simulink model "QZSFuzzy"  (R2017a)
settings: Solver=ode23tb  StartTime=0.0  StopTime=.04  MaxStep=5e-6  RelTol=1e-3  EnableMultiTasking=on
libraries: powerlib x34, simulink x6, fuzblock x1
settings Model: Creator=acer  LastModifiedBy=acer
settings DataIOCC: LimitDataPoints=on  SaveFormat=Array
settings OptimizationCC: LifeSpan=inf
settings DebuggingCC: SFUnexpectedBacktrackingDiag=warning  SFNoUnconditionalDefaultTransitionDiag=warning  SFExecutionAtInitializationDiag=none
settings HardwareCC: ProdBitPerPointer=32  ProdBitPerSizeT=32  ProdBitPerPtrDiffT=32  ProdLargestAtomicFloat=None  ProdIntDivRoundTo=Undefined  ProdEndianess=Unspecified  ProdWordSize=32  ProdHWDeviceType=32-bit Generic
settings ModelReferenceCC: PropagateSignalLabelsOutOfModel=off
settings GRTTargetCC: TargetLangStandard=C89/C90 (ANSI)  GeneratePreprocessorConditionals=Disable all
settings ConfigComp: CovMetricSettings=dw  CovHtmlReporting=on  CovSaveCumulativeToWorkspaceVar=on  CovSaveSingleToWorkspaceVar=on  CovExternalEMLEnable=off

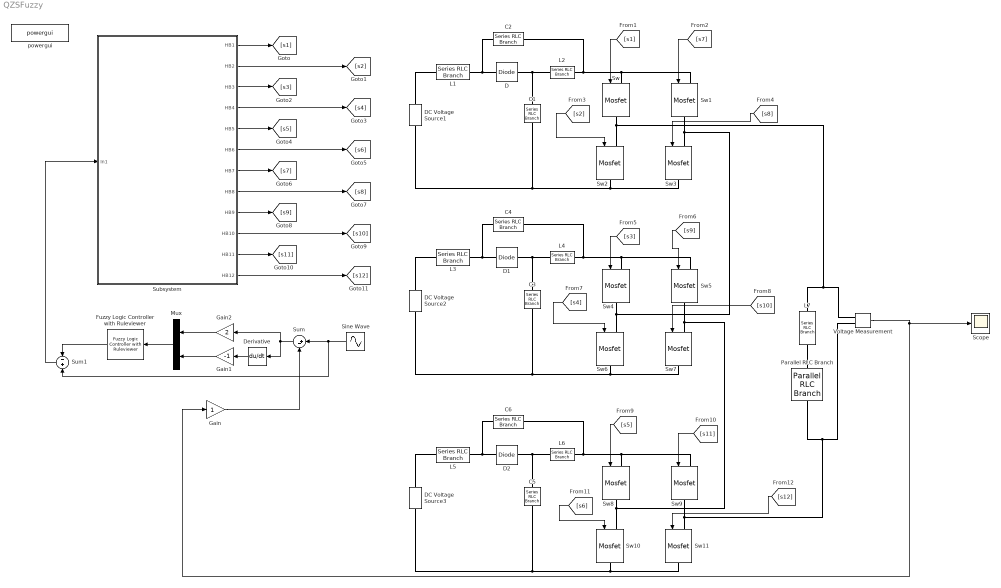
== system QZSFuzzy ==
  C1 : powerlib/Elements/Series RLC Branch  LConnTagsString=__new0  RConnTagsString=__new0  BranchType=C  Resistance=100  Inductance=1e-3  SetiL0=off  InitialCurrent=0  Capacitance=1000e-6  Setx0=off  InitialVoltage=0  Measurements=None
  C2 : powerlib/Elements/Series RLC Branch  LConnTagsString=__new0  RConnTagsString=__new0  BranchType=C  Resistance=1  Inductance=1e-3  SetiL0=off  InitialCurrent=0  Capacitance=1000e-6  Setx0=off  InitialVoltage=0  Measurements=None
  C3 : powerlib/Elements/Series RLC Branch  LConnTagsString=__new0  RConnTagsString=__new0  BranchType=C  Resistance=100  Inductance=1e-3  SetiL0=off  InitialCurrent=0  Capacitance=1000e-6  Setx0=off  InitialVoltage=0  Measurements=None
  C4 : powerlib/Elements/Series RLC Branch  LConnTagsString=__new0  RConnTagsString=__new0  BranchType=C  Resistance=1  Inductance=1e-3  SetiL0=off  InitialCurrent=0  Capacitance=1000e-6  Setx0=off  InitialVoltage=0  Measurements=None
  C5 : powerlib/Elements/Series RLC Branch  LConnTagsString=__new0  RConnTagsString=__new0  BranchType=C  Resistance=100  Inductance=1e-3  SetiL0=off  InitialCurrent=0  Capacitance=1000e-6  Setx0=off  InitialVoltage=0  Measurements=None
  C6 : powerlib/Elements/Series RLC Branch  LConnTagsString=__new0  RConnTagsString=__new0  BranchType=C  Resistance=1  Inductance=1e-3  SetiL0=off  InitialCurrent=0  Capacitance=1000e-6  Setx0=off  InitialVoltage=0  Measurements=None
  D : powerlib/Power Electronics/Diode  Ron=0.001  Lon=0  Vf=.05  IC=0  UseSnubber=off  Rs=500  Cs=250e-9  Measurements=off
  D1 : powerlib/Power Electronics/Diode  Ron=0.001  Lon=0  Vf=.05  IC=0  UseSnubber=off  Rs=500  Cs=250e-9  Measurements=off
  D2 : powerlib/Power Electronics/Diode  Ron=0.001  Lon=0  Vf=.05  IC=0  UseSnubber=off  Rs=500  Cs=250e-9  Measurements=off
  DC Voltage Source1 : powerlib/Electrical Sources/DC Voltage Source  Amplitude=15  Measurements=None
  DC Voltage Source2 : powerlib/Electrical Sources/DC Voltage Source  Amplitude=15  Measurements=None
  DC Voltage Source3 : powerlib/Electrical Sources/DC Voltage Source  Amplitude=15  Measurements=None
  Derivative : Derivative
  Fuzzy Logic Controller with Ruleviewer : fuzblock/Fuzzy Logic  Controller  with Ruleviewer  fismatrix=zsourceRules  Ts=2
  Gain : Gain
  Gain1 : Gain  Gain=-1
  Gain2 : Gain  Gain=2
  L{1..6} (6 alike) : powerlib/Elements/Series RLC Branch  LConnTagsString=__new0  RConnTagsString=__new0  BranchType=L  Resistance=1  Inductance=160e-6  SetiL0=off  InitialCurrent=0  Capacitance=1e-6  Setx0=off  InitialVoltage=0  Measurements=None
  L7 : powerlib/Elements/Series RLC Branch  LConnTagsString=__new0  RConnTagsString=__new0  BranchType=L  Resistance=1  Inductance=100e-3  SetiL0=off  InitialCurrent=0  Capacitance=1e-6  Setx0=off  InitialVoltage=0  Measurements=None
  Mux : Mux  Inputs=2
  Parallel RLC Branch : powerlib/Elements/Parallel RLC Branch  LConnTagsString=a  RConnTagsString=__new0  BranchType=R  Resistance=24  Inductance=1e-3  SetiL0=off  InitialCurrent=0  Capacitance=1e-6  Setx0=off  InitialVoltage=0  Measurements=None
  Scope : Scope
  Sine Wave : Sin  Amplitude=3  Bias=.5  Frequency=2*pi*50  SampleTime=0  VectorParams1D=off
  Subsystem : Subsystem
  Sum : Sum  Inputs=|+-
  Sum1 : Sum  Inputs=-+
  Sw{,1..11} (12 alike) : powerlib/Power Electronics/Mosfet  Ron=0.1  Lon=0  Rd=0.01  Vfd=0  IC=0  Rs=1e5  Cs=inf  Measurements=off
  Voltage Measurement : powerlib/Measurements/Voltage Measurement  PhasorSimulation=off  OutputType=Complex  PSBequivalent=0
  powergui : powerlib/powergui  Priority=1  SimulationMode=Discrete  SampleTime=10e-6  frequency=60  Iterations=50  frequencyindice=0  Pbase=100e6  ErrMax=1e-4  UnitsV=kV  UnitsW=MW  buscounter=0  FunctionMessages=off  echomessages=off  EnableUseOfTLC=off  CurrentSourceSwitches=off  DisableSnubberDevices=off  DisableRonSwitches=off  DisableVfSwitches=off  DisplayEquations=off  SolverType=Tustin/Backward Euler (TBE)  Interpol=off  ExternalGateDelay=off  methode=off  Ts=0  x0status=blocks  SPID=off  SwTol=0  HookPort=off  RestoreLinks=warning  ResistiveCurrentMeasurement=off  Frange=[0:2:500]  Ylog=off  Xlog=on  ShowGrid=off  save=off  variable=ZData  structure=outputVoltage  ZoomFFT=off  StartTime=0.0  cycles=1  DisplayStyle=1  fundamental=60  FreqAxis=off  MaxFrequency=1000  frequencyindicesteady=1  RmsSteady=1  display=off
  wires:
  Voltage Measurement/1 -> Gain/1, Scope/1
  Sine Wave/1 -> Sum1/2, Sum/1
  Gain/1 -> Sum/2
  Sum/1 -> Gain2/1, Derivative/1
  Gain1/1 -> Mux/2
  Gain2/1 -> Mux/1
  Derivative/1 -> Gain1/1
  Mux/1 -> Fuzzy Logic Controller with Ruleviewer/1
  Fuzzy Logic Controller with Ruleviewer/1 -> Sum1/1
  Sum1/1 -> Subsystem/1(In1)
  [s1] -> Sw/1
  [s7] -> Sw1/1
  [s2] -> Sw2/1
  [s8] -> Sw3/1
  [s3] -> Sw4/1
  [s9] -> Sw5/1
  [s10] -> Sw7/1
  [s4] -> Sw6/1
  [s5] -> Sw8/1
  [s11] -> Sw9/1
  [s12] -> Sw11/1
  [s6] -> Sw10/1
  Subsystem/8(HB8) -> [s8]
  Subsystem/1(HB1) -> [s1]
  Subsystem/3(HB3) -> [s3]
  Subsystem/2(HB2) -> [s2]
  Subsystem/9(HB9) -> [s9]
  Subsystem/7(HB7) -> [s7]
  Subsystem/12(HB12) -> [s12]
  Subsystem/4(HB4) -> [s4]
  Subsystem/11(HB11) -> [s11]
  Subsystem/6(HB6) -> [s6]
  Subsystem/5(HB5) -> [s5]
  Subsystem/10(HB10) -> [s10]
  connections:
  L1/RConn1 -- C2/RConn1 -- D/LConn1
  D/RConn1 -- C1/LConn1 -- L2/RConn1
  C2/LConn1 -- Sw1/LConn1 -- Sw/LConn1 -- L2/LConn1
  DC Voltage Source1/RConn1 -- L1/LConn1
  Sw3/RConn1 -- Sw2/RConn1 -- C1/RConn1 -- DC Voltage Source1/LConn1
  L3/RConn1 -- C4/RConn1 -- D1/LConn1
  D1/RConn1 -- C3/LConn1 -- L4/RConn1
  C4/LConn1 -- Sw5/LConn1 -- Sw4/LConn1 -- L4/LConn1
  Sw7/RConn1 -- Sw6/RConn1 -- C3/RConn1 -- DC Voltage Source2/LConn1
  DC Voltage Source2/RConn1 -- L3/LConn1
  Sw1/RConn1 -- Sw6/LConn1 -- Sw4/RConn1 -- Sw3/LConn1
  L5/RConn1 -- C6/RConn1 -- D2/LConn1
  D2/RConn1 -- C5/LConn1 -- L6/RConn1
  C6/LConn1 -- Sw9/LConn1 -- Sw8/LConn1 -- L6/LConn1
  Sw11/RConn1 -- Sw10/RConn1 -- C5/RConn1 -- DC Voltage Source3/LConn1
  DC Voltage Source3/RConn1 -- L5/LConn1
  Sw9/RConn1 -- Voltage Measurement/LConn2 -- Parallel RLC Branch/RConn1 -- Sw11/LConn1
  Sw5/RConn1 -- Sw10/LConn1 -- Sw8/RConn1 -- Sw7/LConn1
  Sw/RConn1 -- L7/LConn1 -- Voltage Measurement/LConn1 -- Sw2/LConn1
  L7/RConn1 -- Parallel RLC Branch/LConn1

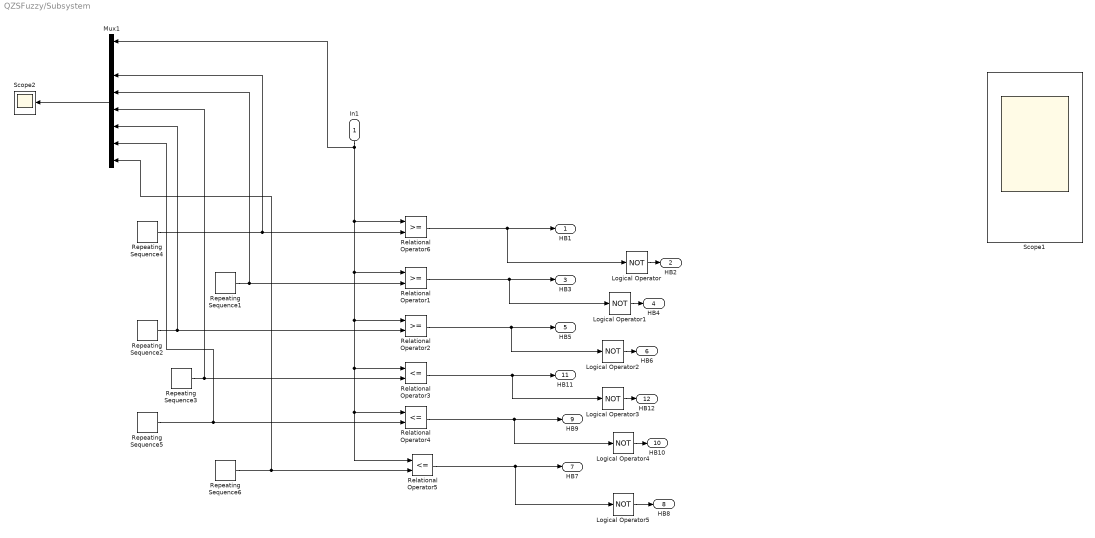
== system QZSFuzzy/Subsystem ==
  In1 : Inport
  Logical Operator{,1..5} (6 alike) : Logic  Operator=NOT  AllPortsSameDT=off  OutDataTypeStr=boolean
  Mux1 : Mux  Inputs=8
  Relational Operator1 : RelationalOperator  OutDataTypeStr=boolean  RndMeth=Nearest
  Relational Operator2 : RelationalOperator  OutDataTypeStr=boolean  RndMeth=Nearest
  Relational Operator3 : RelationalOperator  Operator=<=  OutDataTypeStr=boolean  RndMeth=Nearest
  Relational Operator4 : RelationalOperator  Operator=<=  OutDataTypeStr=boolean  RndMeth=Nearest
  Relational Operator5 : RelationalOperator  Operator=<=  OutDataTypeStr=boolean  RndMeth=Nearest
  Relational Operator6 : RelationalOperator  OutDataTypeStr=boolean  RndMeth=Nearest
  Repeating Sequence1 : simulink/Sources/Repeating Sequence  rep_seq_t="[0  .05e-3  .1e-3]"  rep_seq_y=[1 2 1]
  Repeating Sequence2 : simulink/Sources/Repeating Sequence  rep_seq_t="[0  .05e-3  .1e-3]"  rep_seq_y=[0 1 0]
  Repeating Sequence3 : simulink/Sources/Repeating Sequence  rep_seq_t="[0  .05e-3  .1e-3]"  rep_seq_y=[-1 0 -1]
  Repeating Sequence4 : simulink/Sources/Repeating Sequence  rep_seq_t="[0  .05e-3  .1e-3]"  rep_seq_y=[2 3 2]
  Repeating Sequence5 : simulink/Sources/Repeating Sequence  rep_seq_t="[0  .05e-3  .1e-3]"  rep_seq_y=[-2 -1 -2]
  Repeating Sequence6 : simulink/Sources/Repeating Sequence  rep_seq_t="[0  .05e-3  .1e-3]"  rep_seq_y=[-3 -2 -3]
  Scope1 : Scope  NumInputPorts=7
  Scope2 : Scope
  HB1 : Outport
  HB2 : Outport  Port=2
  HB3 : Outport  Port=3
  HB4 : Outport  Port=4
  HB5 : Outport  Port=5
  HB6 : Outport  Port=6
  HB7 : Outport  Port=7
  HB8 : Outport  Port=8
  HB9 : Outport  Port=9
  HB10 : Outport  Port=10
  HB11 : Outport  Port=11
  HB12 : Outport  Port=12
  wires:
  Relational Operator6/1 -> Logical Operator/1, HB1/1
  Repeating Sequence3/1 -> Relational Operator3/2, Mux1/5
  In1/1 -> Mux1/1, Relational Operator6/1, Relational Operator4/1, Relational Operator5/1, Relational Operator3/1, Relational Operator2/1, Relational Operator1/1
  Repeating Sequence5/1 -> Mux1/7, Relational Operator4/2
  Repeating Sequence2/1 -> Mux1/6, Relational Operator2/2
  Repeating Sequence1/1 -> Mux1/4, Relational Operator1/2
  Repeating Sequence4/1 -> Mux1/3, Relational Operator6/2
  Logical Operator/1 -> HB2/1
  Logical Operator1/1 -> HB4/1
  Relational Operator1/1 -> HB3/1, Logical Operator1/1
  Relational Operator2/1 -> Logical Operator2/1, HB5/1
  Logical Operator2/1 -> HB6/1
  Relational Operator3/1 -> HB11/1, Logical Operator3/1
  Logical Operator3/1 -> HB12/1
  Relational Operator4/1 -> HB9/1, Logical Operator4/1
  Logical Operator4/1 -> HB10/1
  Relational Operator5/1 -> Logical Operator5/1, HB7/1
  Logical Operator5/1 -> HB8/1
  Mux1/1 -> Scope2/1
  Repeating Sequence6/1 -> Mux1/8, Relational Operator5/2
